simulink library "comminteg2"  (Simulink 5.0)
libraries: dspsigattribs x11, commblksprivate x4
settings Model: CovMetricSettings=d  Creator=tdelve  LastModifiedBy=arodrigu  ExtModeAutoUpdateStatusClock=off

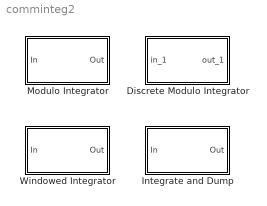
== system comminteg2 ==
  Discrete Modulo Integrator : Subsystem  mask(Discrete Modulo Integrator){method=Forward Euler, modu=1, init=0, ts=1}
      mask prompts: method "Integration method:"; modu "Absolute value bound:"; init "Initial condition:"; ts "Sample time:"
      mask help:
      | Integrate the input signal in discrete time and then uses the Absolute value bound parameter, K, to produce output strictly between -K and K. The block uses the rem function in MATLAB.
      |
      | The input can be either a scalar, a sample-based vector, or a frame-based row vector.  This block processes each vector element independently.
      mask init:
      | commblkdmodint(gcb);
      settings: ErrorFcn=commblkdmint
      mask Help: helpview(commbhelp)
      mask StyleString: popup(Forward Euler|Backward Euler|Trapezoidal),edit,edit,edit
      mask Display: disp('Discrete\nModulo\nIntegrator')
  Integrate and Dump : Subsystem  mask(Integrate and Dump){limit=1, td=2, ts=1}
      mask prompts: limit "Absolute value bound:"; td "Integration period (s):"; ts "Sample time:"
      mask help:
      | Integrate the input signal in discrete time over the Integration period and then reduce modulo the Absolute value bound parameter. The integrator resets its internal state before integrating the next period.
      |
      | The input can be either a scalar, a sample-based vector, or a frame-based row vector.  This block processes each vector element independently.
      mask init:
      | limit(find(isinf(limit))) = realmax;
      | td(find(isinf(td))) = realmax;
      | 
      | if(~isempty(ts))
      |    if(length(ts) ~= 1)
      |       error('Sample time parameter must be a real scalar.');
      |    end;
      | end;
      settings: ErrorFcn=commblkintdmp
      mask Help: helpview(commbhelp)
      mask Display: disp('Integrate\nand Dump')
  Modulo Integrator : Subsystem  mask(Modulo Integrator){modu=1, init=0}
      mask prompts: modu "Absolute value bound:"; init "Initial condition:"
      mask help:
      | Integrate the input signal in continuous time and then uses the Absolute value bound parameter, K, to produce output strictly between -K and K. The block uses the rem function in MATLAB.
      |
      | The input must be sample-based.
      mask init:
      | [modu, init]=commblkmodint(gcb);
      mask Help: helpview(commbhelp)
      mask Display: disp('Modulo\nIntegrator')
  Windowed Integrator : Subsystem  mask(Windowed Integrator){method=Forward Euler, vec=1, T=2, sample_time=1}
      mask prompts: method "Integration method:"; vec "Input vector size:"; T "Integration window length (s):"; sample_time "Sample time:"
      mask help:
      | Integrate the input signal in discrete time from time t-T to t where T is the Integration window length. This block assumes that the signal is zero for all negative times.
      |
      | The input can be either a scalar, a sample-based vector, or a frame-based row vector.  This block processes each vector element independently.
      mask init:
      | method = lower(method);
      | 
      | switch method
      | case {'forward euler' 'backward euler'}
      | case 'trapezoidal'
      | 	method = 'first order';
      | otherwise
      |    error('Unknown integration method.')
      | end;
      | 
      | if(~isempty(sample_time))
      |    if(length(sample_time) ~= 1)
      |       error('Sample time parameter must be a real scalar.');
      |    end;
      | end;
      settings: ErrorFcn=commblkwint
      mask Help: helpview(commbhelp)
      mask StyleString: popup(Forward Euler|Backward Euler|Trapezoidal),edit,edit,edit
      mask Display: disp('Windowed\nIntegrator')

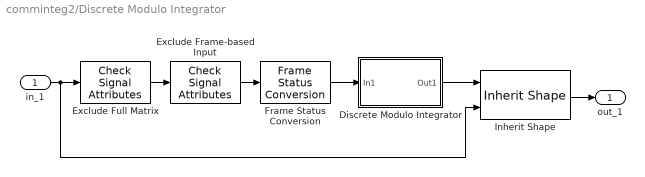
== system comminteg2/Discrete Modulo Integrator ==
  in_1 : Inport
  Discrete Modulo Integrator : Subsystem
  "Exclude Frame-based Input " : dspsigattribs/Check Signal Attributes  SigAttribCheckMethod=Matches attributes exactly  Complexity=Ignore  Frame=Frame-based  DimsCheckMethod=Is not...  Dimensions=Row vector (2-D) or scalar  DatatypeCheckMethod=Ignore  DatatypeGeneral=Boolean  DtypeFloatSpecific=Any floating-point  DtypeFixedSpecific=Any fixed-point  DtypeIntSpecific=Any integer  SampleMode=Ignore
  Exclude Full Matrix : dspsigattribs/Check Signal Attributes  SigAttribCheckMethod=Matches attributes exactly  Complexity=Ignore  Frame=Ignore  DimsCheckMethod=Is...  Dimensions=Full matrix (2-D)  DatatypeCheckMethod=Ignore  DatatypeGeneral=Boolean  DtypeFloatSpecific=Any floating-point  DtypeFixedSpecific=Any fixed-point  DtypeIntSpecific=Any integer  SampleMode=Ignore
  Frame Status Conversion : dspsigattribs/Frame Status Conversion  growRefPort=off  outframe=Sample-based
  Inherit Shape : commblksprivate/Inherit Shape
  out_1 : Outport  InitialOutput=0
  wires:
  in_1/1 -> Exclude Full Matrix/1, Inherit Shape/2
  Inherit Shape/1 -> out_1/1
  Exclude Full Matrix/1 -> "Exclude Frame-based Input "/1
  "Exclude Frame-based Input "/1 -> Frame Status Conversion/1
  Frame Status Conversion/1 -> Discrete Modulo Integrator/1(In1)
  Discrete Modulo Integrator/1(Out1) -> Inherit Shape/1

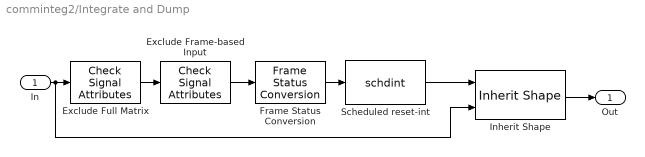
== system comminteg2/Integrate and Dump ==
  In : Inport
  "Exclude Frame-based Input " : dspsigattribs/Check Signal Attributes  SigAttribCheckMethod=Matches attributes exactly  Complexity=Ignore  Frame=Frame-based  DimsCheckMethod=Is not...  Dimensions=Row vector (2-D) or scalar  DatatypeCheckMethod=Ignore  DatatypeGeneral=Boolean  DtypeFloatSpecific=Any floating-point  DtypeFixedSpecific=Any fixed-point  DtypeIntSpecific=Any integer  SampleMode=Ignore
  Exclude Full Matrix : dspsigattribs/Check Signal Attributes  SigAttribCheckMethod=Matches attributes exactly  Complexity=Ignore  Frame=Ignore  DimsCheckMethod=Is...  Dimensions=Full matrix (2-D)  DatatypeCheckMethod=Ignore  DatatypeGeneral=Boolean  DtypeFloatSpecific=Any floating-point  DtypeFixedSpecific=Any fixed-point  DtypeIntSpecific=Any integer  SampleMode=Ignore
  Frame Status Conversion : dspsigattribs/Frame Status Conversion  growRefPort=off  outframe=Sample-based
  Inherit Shape : commblksprivate/Inherit Shape
  Scheduled reset-int : S-Function  FunctionName=schdint  Parameters=td, ts, limit
  Out : Outport  InitialOutput=0
  wires:
  In/1 -> Exclude Full Matrix/1, Inherit Shape/2
  Scheduled reset-int/1 -> Inherit Shape/1
  Inherit Shape/1 -> Out/1
  Frame Status Conversion/1 -> Scheduled reset-int/1
  "Exclude Frame-based Input "/1 -> Frame Status Conversion/1
  Exclude Full Matrix/1 -> "Exclude Frame-based Input "/1

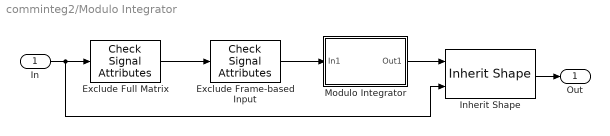
== system comminteg2/Modulo Integrator ==
  In : Inport
  "Exclude Frame-based Input " : dspsigattribs/Check Signal Attributes  SigAttribCheckMethod=Matches attributes exactly  Complexity=Ignore  Frame=Frame-based  DimsCheckMethod=Ignore  Dimensions=Scalar (1-D or 2-D)  DatatypeCheckMethod=Ignore  DatatypeGeneral=Boolean  DtypeFloatSpecific=Any floating-point  DtypeFixedSpecific=Any fixed-point  DtypeIntSpecific=Any integer  SampleMode=Ignore
  Exclude Full Matrix : dspsigattribs/Check Signal Attributes  SigAttribCheckMethod=Matches attributes exactly  Complexity=Ignore  Frame=Ignore  DimsCheckMethod=Is...  Dimensions=Full matrix (2-D)  DatatypeCheckMethod=Ignore  DatatypeGeneral=Boolean  DtypeFloatSpecific=Any floating-point  DtypeFixedSpecific=Any fixed-point  DtypeIntSpecific=Any integer  SampleMode=Ignore
  Inherit Shape : commblksprivate/Inherit Shape
  Modulo Integrator : Subsystem
  Out : Outport
  wires:
  Inherit Shape/1 -> Out/1
  Modulo Integrator/1(Out1) -> Inherit Shape/1
  In/1 -> Inherit Shape/2, Exclude Full Matrix/1
  "Exclude Frame-based Input "/1 -> Modulo Integrator/1(In1)
  Exclude Full Matrix/1 -> "Exclude Frame-based Input "/1

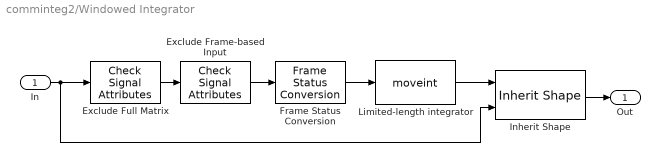
== system comminteg2/Windowed Integrator ==
  In : Inport
  "Exclude Frame-based Input " : dspsigattribs/Check Signal Attributes  SigAttribCheckMethod=Matches attributes exactly  Complexity=Ignore  Frame=Frame-based  DimsCheckMethod=Is not...  Dimensions=Row vector (2-D) or scalar  DatatypeCheckMethod=Ignore  DatatypeGeneral=Boolean  DtypeFloatSpecific=Any floating-point  DtypeFixedSpecific=Any fixed-point  DtypeIntSpecific=Any integer  SampleMode=Ignore
  Exclude Full Matrix : dspsigattribs/Check Signal Attributes  SigAttribCheckMethod=Matches attributes exactly  Complexity=Ignore  Frame=Ignore  DimsCheckMethod=Is...  Dimensions=Full matrix (2-D)  DatatypeCheckMethod=Ignore  DatatypeGeneral=Boolean  DtypeFloatSpecific=Any floating-point  DtypeFixedSpecific=Any fixed-point  DtypeIntSpecific=Any integer  SampleMode=Ignore
  Frame Status Conversion : dspsigattribs/Frame Status Conversion  growRefPort=off  outframe=Sample-based
  Inherit Shape : commblksprivate/Inherit Shape
  Limited-length integrator : S-Function  FunctionName=moveint  Parameters=vec,T,sample_time,method
  Out : Outport  InitialOutput=0
  wires:
  In/1 -> Exclude Full Matrix/1, Inherit Shape/2
  Limited-length integrator/1 -> Inherit Shape/1
  Inherit Shape/1 -> Out/1
  Exclude Full Matrix/1 -> "Exclude Frame-based Input "/1
  "Exclude Frame-based Input "/1 -> Frame Status Conversion/1
  Frame Status Conversion/1 -> Limited-length integrator/1

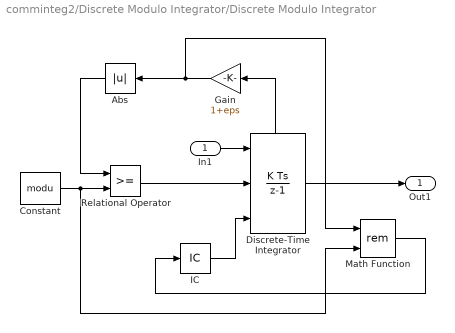
== system comminteg2/Discrete Modulo Integrator/Discrete Modulo Integrator ==
  In1 : Inport
  Abs : Abs  Orientation=left  SaturateOnIntegerOverflow=on
  Constant : Constant  Value=modu
  Discrete-Time Integrator : DiscreteIntegrator  ExternalReset=rising  InitialConditionSource=external  UpperSaturationLimit=2*modu  LowerSaturationLimit=-2*modu  ShowStatePort=on  SampleTime=ts
  Gain : Gain  Orientation=left  Gain=1+eps  SaturateOnIntegerOverflow=on
  IC : InitialCondition  Value=init
  Math Function : Math  Operator=rem
  Relational Operator : RelationalOperator  InputSameDT=on
  Out1 : Outport
  wires:
  IC/1 -> Discrete-Time Integrator/3
  Discrete-Time Integrator/1 -> Out1/1
  Math Function/1 -> IC/1
  Relational Operator/1 -> Discrete-Time Integrator/2
  Discrete-Time Integrator/State -> Gain/1
  Abs/1 -> Relational Operator/1
  Constant/1 -> Math Function/2, Relational Operator/2
  In1/1 -> Discrete-Time Integrator/1
  Gain/1 -> Abs/1, Math Function/1

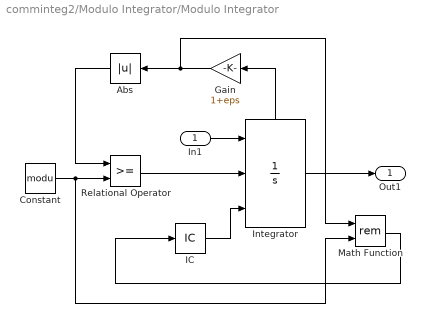
== system comminteg2/Modulo Integrator/Modulo Integrator ==
  In1 : Inport
  Abs : Abs  Orientation=left  SaturateOnIntegerOverflow=on
  Constant : Constant  Value=modu
  Gain : Gain  Orientation=left  Gain=1+eps  SaturateOnIntegerOverflow=on
  IC : InitialCondition  Value=init
  Integrator : Integrator  ExternalReset=rising  InitialConditionSource=external  UpperSaturationLimit=1  LowerSaturationLimit=0  ShowStatePort=on
  Math Function : Math  Operator=rem
  Relational Operator : RelationalOperator  InputSameDT=on
  Out1 : Outport
  wires:
  Gain/1 -> Math Function/1, Abs/1
  Integrator/State -> Gain/1
  Constant/1 -> Relational Operator/2, Math Function/2
  Relational Operator/1 -> Integrator/2
  Abs/1 -> Relational Operator/1
  Math Function/1 -> IC/1
  Integrator/1 -> Out1/1
  In1/1 -> Integrator/1
  IC/1 -> Integrator/3
